simulink model "DCAC_conv_GFM"  (R2025a)
settings: Solver=VariableStepAuto  StartTime=0.0  StopTime=10.0  RelTol=1e-3
undefined symbols (not defined in the file): block_buses_DC, block_idx, Grid_op_VCVSC, Kic, Kiv, Kpc, Kpv, Nbuses_DC, op_VCVSC
libraries: simulink x6
(part 1 of 2)
settings Model: Creator=atomas  LastModifiedBy=atomas

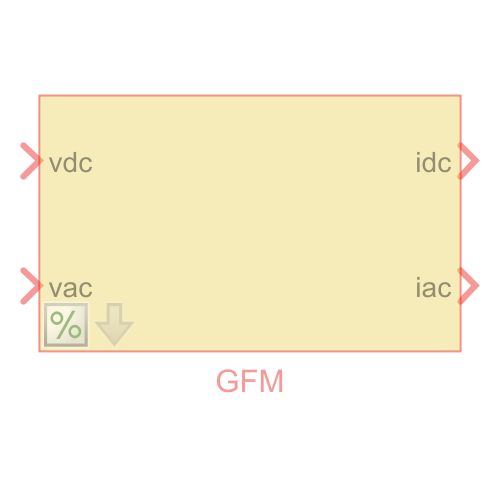
[thumbnail: Simulink's stored preview of the top-level diagram]
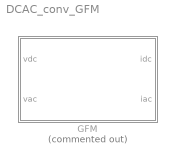
== system DCAC_conv_GFM ==
  GFM : Subsystem  Commented=on  mask(VCVSC){Pmax=Inf, Qmax=Inf, fb=50, dynamic_VCC=Static, Lf=0.01, Rf=0.001, Rcf=1000000, Cfi=0.1, Kint=1, Tint=0.1, Bint=1, Kext=1, Bext=1, Text=0.1, Fi=1, Tf=0.01, mp=0.01, nq=0.01, VI_L=0.1, VI_R=0.01, WOF_Tf=0, cf=0.1, cv=0.1, L_out=0.1, R_out=0.01}
      mask prompts: Pmax "Active power limit (p.u.)"; Qmax "Reactive power limit (p.u.)"; fb "Base frequency (Hz)"; dynamic_VCC "Dynamic behavior"; Lf "Filter inductance (pu)"; Rf "Filter resistance (pu)"; Rcf "Parallel resistance to C (pu)"; Cfi "Filter capacitance (pu)"; Fi "Current feedfordward gain"; Tf "Low-pass filter time constant (s)"; mp "Droop coefficient mp (pu)"; nq "Droop coefficient nq (pu)"; VI_L "Inductance (pu)"; VI_R "Resistance (pu)"; WOF_Tf "WOF time constant (s)"; cf "Frequency SC gain"; cv "Voltage SC gain"; L_out "Output inductance (p.u.)"; R_out "Output resistance (p.u.)"
      mask help: Grid-forming converter. VCC are the voltage and current controllers. Dynamic behavior includes the PI controllers, decoupling, current feedfordward and LC output filter. Static behavior consists of setting the reference voltage directly in the output. PC is the power controller including the droop control and low-pass filters for the power measurements.
      mask init:
      | mdlWks = get_param(bdroot,'ModelWorkspace'); % Get the model workspace
      | block_name = get_param(gcb,'Name');
      | bvarname = get_param(get_param(get_param(get_param(...
      |         gcb, 'Parent'), 'Parent'), 'Parent'), 'bvarname');
      | DC = mdlWks.getVariable([bvarname 'DC']);
      | try
      |     block_DC_buses = DC.(block_name + "s_DC_buses");
      |     block_buses = DC.(block_name + "s_buses");
      |     block_DC_toM = DC.(block_name + "s_DC_toM");
      |     block_toM = DC.(block_name + "s_toM");
      |     dparams = DC.(block_name + "_dparams");
      | catch ME
      |     %errordlg(ME.message)
      | end
      mask Help: web('Documentation/VCVSC.html')
      mask TypeOptions dynamic_VCC: Dynamic with limitation | Dynamic | Static | Dynamic VC and static CC
      mask Callback dynamic_VCC:
      | block = gcb;
      | dynamic = get_param(block, 'dynamic_VCC');
      | param_vis = get_param(block,'MaskVisibilities');
      | block_params = string(fieldnames(get_param(block, 'DialogParameters')));
      | switch dynamic
      |     case 'Dynamic'
      |         param_vis(find(block_params == 'Lf'):find(block_params == 'Fi')) = cellstr("on");
      |         set_param([gcb '/VCC'], 'LabelModeActiveChoice', 'dynamic');
      |     case 'Dynamic with limitation'
      |         param_vis(find(block_params == 'Lf'):find(block_params == 'Fi')) = cellstr("on");
      |         set_param([gcb '/VCC'], 'LabelModeActiveChoice', 'dynamic_limiting');
      |     case 'Static'
      |         param_vis(find(block_params == 'Lf'):find(block_params == 'Fi')) = cellstr("off");
      |         set_param([gcb '/VCC'], 'LabelModeActiveChoice', 'static');
      |     case 'Dynamic VC and static CC'
      |         param_vis(find(block_params == 'Lf'):find(block_params == 'Fi')) = cellstr("on");
      |         param_vis(ismember(block_params, ["Lf","Rf","Kpc","Kic","Fi"])) = cellstr("off");
      |         set_param([gcb '/VCC'], 'LabelModeActiveChoice', 'dynamic_VC');
      | end
      | set_param(block,'MaskVisibilities',param_vis)
      mask TypeOptions Tf: PC/Tf
      mask TypeOptions mp: PC/mp
      mask TypeOptions nq: PC/nq
      mask TypeOptions VI_L: VI/L
      mask TypeOptions VI_R: VI/R
      mask TypeOptions WOF_Tf: VI/Tf
      mask DialogControl Container8 Prompt: Parameters
      mask DialogControl VCC Prompt: VCC
      mask DialogControl PC Prompt: PC
      mask DialogControl VI Prompt: VI
      mask DialogControl SC Prompt: SC
      mask DialogControl Container9 Prompt: Others

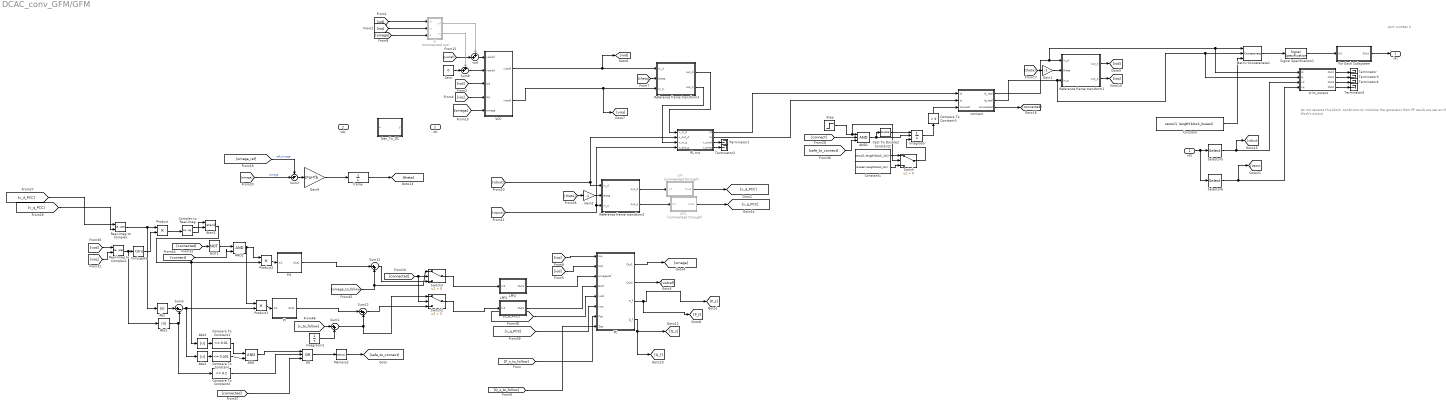
== system DCAC_conv_GFM/GFM ==
  note: do not rename this block, conditions to initialise the generator from PF result are set on this block's output
  note: port number 2
  vac : Inport
  vdc : Inport  Port=2
  AND : Logic  IconShape=distinctive  AllPortsSameDT=off  OutDataTypeStr=boolean
  AND1 : Logic  Inputs=3  IconShape=distinctive  AllPortsSameDT=off  OutDataTypeStr=boolean
  AND2 : Logic  IconShape=distinctive  AllPortsSameDT=off  OutDataTypeStr=boolean
  Abs{,1..3} (4 alike) : Abs  ZeroCross=off  SaturateOnIntegerOverflow=off
  Atan2 : Trigonometry  Operator=atan2
  Cast To Double2 : DataTypeConversion  OutDataTypeStr=double  SaturateOnIntegerOverflow=off  RndMeth=Floor
  Compare To Constant : simulink/Logic and Bit Operations/Compare To Constant  relop=<=  const=0.001  OutDataTypeStr=boolean  ZeroCross=off
  Compare To Constant1 : simulink/Logic and Bit Operations/Compare To Constant  relop=<=  const=0.01  OutDataTypeStr=boolean  ZeroCross=off
  Compare To Constant2 : simulink/Logic and Bit Operations/Compare To Constant  relop=<=  const=0.2  OutDataTypeStr=boolean  ZeroCross=off
  Compare To Constant3 : simulink/Logic and Bit Operations/Compare To Constant  relop=>  const=4  OutDataTypeStr=boolean  ZeroCross=off
  Complex to Real-Imag : ComplexToRealImag
  Conjugate : Math  Operator=conj  SignedPower=on  RndMeth=Zero
  Constant : Constant  Value=zeros(1, length(block_buses))  VectorParams1D=off
  Constant1 : Constant  Value=5*ones(1,length(block_idx))  VectorParams1D=off
  Constant2 : Constant  Value=zeros(1,length(block_idx))  VectorParams1D=off
  For Each Subsystem : Subsystem  TreatAsAtomicUnit=on
  Gain1 : Gain  Gain=-1
  Gain2 : Gain  Gain=-1
  Gain6 : Gain  Gain=2*pi*fb
  Gen_To_DC : MATLAB Function  TreatAsAtomicUnit=on
  Integrator : Integrator  ExternalReset=falling  InitialConditionSource=external  InitialCondition=Grid_op_VCVSC.States(1,:)
  Integrator1 : Integrator  InitialCondition=Grid_op_VCVSC.States(2,:)
  LPF : Subsystem  Commented=through
  LPF1 : Subsystem  Commented=through
  LPF2 : Subsystem
  LPF3 : Subsystem
  Matrix Concatenate1 : Concatenate  NumInputs=3  Mode=Multidimensional array
  Memory2 : Memory  InitialCondition=1
  NOT1 : Logic  Operator=NOT  IconShape=distinctive  AllPortsSameDT=off  OutDataTypeStr=boolean
  OR : Logic  Operator=OR  Inputs=3  IconShape=distinctive  AllPortsSameDT=off  OutDataTypeStr=boolean
  PC : Subsystem  mask(PC_VCVSC){Tf=Tf, mp=mp, nq=nq}
      mask prompts: Tf "Low-pass filter time constant (s)"; mp "Droop coefficient mp"; nq "Droop coefficient nq"
      mask help: Power controller of a grid-forming converter, including the droop control and low-pass filters for the power measurements.
      mask init:
      | if all(Tf ~= 0)
      |     iTf = 1./Tf;
      |     set_param([gcb '/LPF_P'],'Commented','off')
      |     set_param([gcb '/LPF_Q'],'Commented','off')
      | else
      |     set_param([gcb '/LPF_P'],'Commented','through')
      |     set_param([gcb '/LPF_Q'],'Commented','through')
      | end
  PI : Subsystem
  PI1 : Subsystem
  Product : Product
  Product1 : Product  OutDataTypeStr=double
  Product2 : Product  OutDataTypeStr=double
  RL out : Subsystem  Variant=on  VariantControlMode=label  LabelModeActiveChoice=dynamic  mask{dynamic=Dynamic, R=R_out, L=L_out, fbase=50}
      mask prompts: dynamic "Dynamic behavior"; R "Series resistance (p.u.)"; L "Inductance (p.u.)"; fbase "Base frequency (Hz)"
      mask init:
      | omegab = 2*pi*fbase;
      | invL = 1./L;
      | vssBlk = gcb;
      | switch dynamic
      |     case "Static"
      |         set_param(vssBlk, 'LabelModeActiveChoice', 'static');
      |     case "Dynamic"
      |         set_param(vssBlk, 'LabelModeActiveChoice', 'dynamic');
      |     case "Static omega"
      |         set_param(vssBlk, 'LabelModeActiveChoice', 'static_omega');
      | end
      mask TypeOptions dynamic: Static | Dynamic | Static omega
  Real-Imag to Complex : RealImagToComplex
  Real-Imag to Complex1 : RealImagToComplex
  Reference frame transform1 : Subsystem
  Reference frame transform2 : Subsystem
  Reference frame transform3 : Subsystem
  Selector5 : Selector  NumberOfDimensions=2  InputPortWidth=3  IndexOptions=Index vector (dialog),Index vector (dialog)  Indices=1,block_buses  OutputSizes=1,1
  Selector6 : Selector  NumberOfDimensions=2  InputPortWidth=3  IndexOptions=Index vector (dialog),Index vector (dialog)  Indices=2,block_buses  OutputSizes=1,1
  Signal Specification1 : SignalSpecification  Dimensions=[3 length(block_buses)]
  Step : Step  Time=0.01  SampleTime=0  VectorParams1D=off  ZeroCross=off
  Sum1 : Sum  Inputs=|++
  Sum11 : Sum  Inputs=|++
  Sum12 : Sum  Inputs=|++
  Sum2 : Sum  Inputs=-+|
  Sum3 : Sum  Inputs=|+-
  Sum8 : Sum  Inputs=++|
  Switch : Switch  Criteria=u2 > Threshold  SaturateOnIntegerOverflow=off  InputSameDT=off
  Switch2 : Switch  Criteria=u2 > Threshold  SaturateOnIntegerOverflow=off  InputSameDT=off
  Switch3 : Switch  Criteria=u2 > Threshold  SaturateOnIntegerOverflow=off  InputSameDT=off
  Terminator{,1..5} (6 alike) : Terminator
  VCC : Subsystem  Variant=on  VariantControlMode=label  LabelModeActiveChoice=static
  VI : Subsystem  Commented=on  mask{L=VI_L, R=VI_R, Tf=WOF_Tf}
      mask prompts: L "Inductance (pu)"; R "Resistance (pu)"; Tf "WOF time constant (s)"
      mask init:
      | if all(Tf ~= 0)
      |     iTf = 1./Tf;
      |     set_param([gcb '/WOF_d'],'Commented','off')
      |     set_param([gcb '/WOF_q'],'Commented','off')
      | else
      |     set_param([gcb '/WOF_d'],'Commented','through')
      |     set_param([gcb '/WOF_q'],'Commented','through')
      | end
  Zero : Constant  Value=0  OutDataTypeStr=Inherit: Inherit via back propagation
  connect : Subsystem
  frame : Integrator  InitialCondition=Grid_op_VCVSC.States(19,:)  IgnoreLimit=on
  trim_output : Subsystem
  vod : Sum  Inputs=++|
  iac : Outport
  idc : Outport  Port=2
  wires:
  Sum8/1 -> VCC/2(voqref)
  vod/1 -> VCC/1(vodref)
  [omega] -> VI/3(omega)
  [ioq] -> VI/2(iq)
  [iod] -> VI/1(id)
  Gain2/1 -> Reference frame transform2/2(theta)
  [theta] -> Gain2/1
  Gain6/1 -> frame/1
  frame/1 -> [theta]
  PC/4(Q_f) -> [Q_s], [Q_f]
  PC/3(P_f) -> [P_s], [P_f]
  connect/3(connected) -> [connected]
  [omega] -> Sum2/2  "omega"
  [omega_ref] -> Sum2/1  "ref_omega"
  Sum2/1 -> Gain6/1
  RL out/1(id) -> connect/1(id)
  [theta] -> Gain1/1
  Gain1/1 -> Reference frame transform1/2(theta)
  [ioq] -> VCC/4(ioq)
  [iod] -> VCC/3(iod)
  Zero/1 -> Sum8/2
  [vodref] -> vod/2
  [omega] -> VCC/5(omega)
  [theta] -> Reference frame transform3/2(theta)
  PC/1(Out1) -> [omega]
  PC/2(Out2) -> [vodref]
  [iod] -> PC/2(iodi)
  [ioq] -> PC/1(ioq)
  Reference frame transform1/2(out_q) -> [ioq]
  Reference frame transform3/1(out_d) -> RL out/1(v_in_d)
  Reference frame transform3/2(out_q) -> RL out/3(v_in_q)
  RL out/2(iq) -> connect/2(iq)
  Reference frame transform1/1(out_d) -> [iod]
  VI/1(vd) -> vod/1
  VI/2(vq) -> Sum8/1
  connect/1(id_real) -> trim_output/1(id), Matrix Concatenate1/1, Reference frame transform1/1(in_d)
  connect/2(iq_real) -> trim_output/2(iq), Matrix Concatenate1/2, Reference frame transform1/3(in_q)
  RL out/3(v_outd) -> Terminator1/1
  RL out/4(v_outq) -> Terminator2/1
  Reference frame transform2/1(out_d) -> LPF/1(In1)
  Reference frame transform2/2(out_q) -> LPF1/1(In1)
  [v_d_PCC] -> Real-Imag to Complex/1
  [v_q_PCC] -> Real-Imag to Complex/2
  [vod] -> Real-Imag to Complex1/1
  [voq] -> Real-Imag to Complex1/2
  Real-Imag to Complex1/1 -> Abs1/1, Conjugate/1
  Real-Imag to Complex/1 -> Abs/1, Product/1
  Conjugate/1 -> Product/2
  Product/1 -> Complex to Real-Imag/1
  Complex to Real-Imag/2 -> Atan2/1
  Complex to Real-Imag/1 -> Atan2/2
  Abs/1 -> Sum3/1
  Sum3/1 -> Abs2/1, Product1/2
  Product1/1 -> PI/1(In1)
  Product2/1 -> PI1/1(In1)
  Atan2/1 -> Abs3/1, Product2/2
  Abs1/1 -> Compare To Constant2/1, Sum3/2
  Abs2/1 -> Compare To Constant/1
  Compare To Constant/1 -> AND/2
  Abs3/1 -> Compare To Constant1/1
  Compare To Constant1/1 -> AND/1
  AND/1 -> OR/1
  OR/1 -> Memory2/1
  Compare To Constant2/1 -> OR/2
  [connected] -> OR/3
  Memory2/1 -> [safe_to_connect]
  [vqout] -> Reference frame transform2/3(in_q), RL out/4(v_out_q)
  LPF/1(Out1) -> [v_d_PCC]
  LPF1/1(Out1) -> [v_q_PCC]
  [vdout] -> RL out/2(v_out_d), Reference frame transform2/1(in_d)
  Matrix Concatenate1/1 -> Signal Specification1/1
  Constant/1 -> Matrix Concatenate1/3
  For Each Subsystem/1(Out1) -> iac/1
  Signal Specification1/1 -> For Each Subsystem/1(In1)
  [v_d_PCC] -> PC/5(vodi)
  [v_q_PCC] -> PC/6(voq)
  trim_output/1(Out1) -> Terminator/1
  trim_output/2(Out2) -> Terminator3/1
  trim_output/3(Out3) -> Terminator4/1
  trim_output/4(Out4) -> Terminator5/1
  vac/1 -> Selector6/1, Selector5/1
  Selector6/1 -> [vqout], trim_output/4(vq)
  Selector5/1 -> [vdout], trim_output/3(vd)
  NOT1/1 -> AND2/1
  [connected] -> NOT1/1
  AND2/1 -> Product1/1, Product2/1
  [connect] -> AND1/2
  Integrator/1 -> Compare To Constant3/1
  Constant2/1 -> Switch/1
  Step/1 -> Switch/2, AND1/1
  Constant1/1 -> Switch/3
  [safe_to_connect] -> AND1/3
  AND1/1 -> Cast To Double2/1, Integrator/2
  Cast To Double2/1 -> Integrator/1
  Switch/1 -> Integrator/3
  VCC/1(vidref) -> [vod], Reference frame transform3/1(in_d)
  VCC/2(viqref) -> [voq], Reference frame transform3/3(in_q)
  Sum12/1 -> Switch2/3
  Sum1/1 -> Switch2/1, Sum12/2
  [omega_to_follow] -> Sum11/2, Switch3/1
  [connected] -> Switch2/2, Switch3/2
  PI/1(Out1) -> Sum12/1
  PI1/1(Out1) -> Sum11/1
  Sum11/1 -> Switch3/3
  Switch3/1 -> LPF2/1(In1)
  Switch2/1 -> LPF3/1(In1)
  [P_s_to_follow] -> PC/7(Psp)
  [Q_s_to_follow] -> PC/8(Qsp)
  [v_to_follow] -> Sum1/1
  Integrator1/1 -> Sum1/2
  Compare To Constant3/1 -> connect/3(connect)
  [connect] -> AND2/2
  LPF2/1(Out1) -> PC/3(omegaref)
  LPF3/1(Out1) -> PC/4(Eref)

== system DCAC_conv_GFM/GFM/For Each Subsystem ==
  In1 : Inport  Partition=on  PartitionDimension=1  PartitionWidth=1  PartitionOffset=0
  For Each : ForEach  DisableCoverage=on
  State-Space : StateSpace  A=[]  B=[]  C=[]  D=block_toM  InitialCondition=0  ParameterTunability=Optimized
  Transpose : Math  Operator=transpose
  Transpose1 : Math  Operator=transpose
  Out1 : Outport  ConcatenationDimension=1
  wires:
  State-Space/1 -> Transpose1/1
  Transpose/1 -> State-Space/1
  Transpose1/1 -> Out1/1
  In1/1 -> Transpose/1

== system DCAC_conv_GFM/GFM/LPF ==
  In1 : Inport
  Gain : Gain  Gain=1e2
  I : Integrator  InitialCondition=Grid_op_VCVSC.op.States(4).x'
  Sum4 : Sum  Inputs=|+-
  Out1 : Outport
  wires:
  Gain/1 -> I/1
  Sum4/1 -> Gain/1
  In1/1 -> Sum4/1
  I/1 -> Out1/1, Sum4/2

== system DCAC_conv_GFM/GFM/LPF1 ==
  In1 : Inport
  Gain : Gain  Gain=1e2
  I : Integrator  InitialCondition=Grid_op_VCVSC.op.States(5).x'
  Sum4 : Sum  Inputs=|+-
  Out1 : Outport
  wires:
  I/1 -> Sum4/2, Out1/1
  In1/1 -> Sum4/1
  Sum4/1 -> Gain/1
  Gain/1 -> I/1

== system DCAC_conv_GFM/GFM/LPF2 ==
  In1 : Inport
  Gain : Gain  Gain=1e2
  I : Integrator  InitialCondition=Grid_op_VCVSC.States(3,:)
  Sum4 : Sum  Inputs=|+-
  Out1 : Outport
  wires:
  I/1 -> Sum4/2, Out1/1
  In1/1 -> Sum4/1
  Sum4/1 -> Gain/1
  Gain/1 -> I/1

== system DCAC_conv_GFM/GFM/LPF3 ==
  In1 : Inport
  Gain : Gain  Gain=1e2
  I : Integrator  InitialCondition=Grid_op_VCVSC.States(4,:)
  Sum4 : Sum  Inputs=|+-
  Out1 : Outport
  wires:
  Gain/1 -> I/1
  Sum4/1 -> Gain/1
  In1/1 -> Sum4/1
  I/1 -> Out1/1, Sum4/2

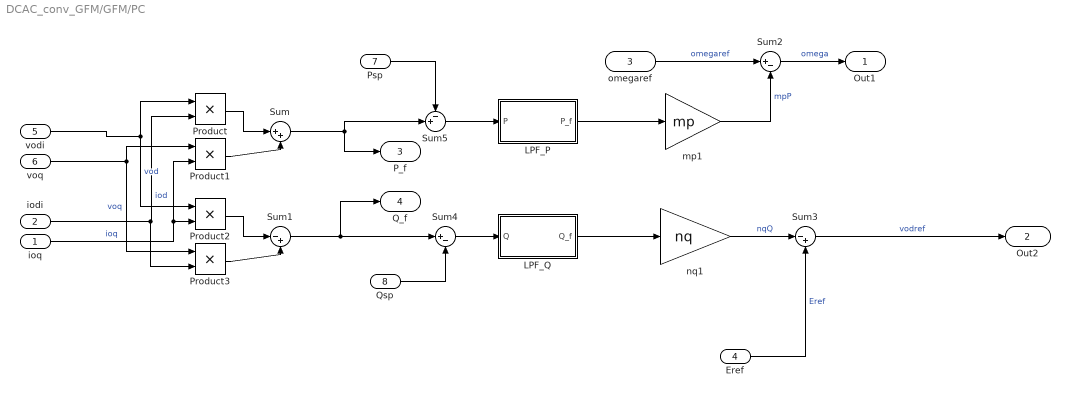
== system DCAC_conv_GFM/GFM/PC ==
  ioq : Inport
  iodi : Inport  Port=2
  omegaref : Inport  Port=3
  Eref : Inport  Port=4
  vodi : Inport  Port=5
  voq : Inport  Port=6
  Psp : Inport  Port=7
  Qsp : Inport  Port=8
  LPF_P : Subsystem
  LPF_Q : Subsystem
  Product{,1..3} (4 alike) : Product
  Sum : Sum  Inputs=|++
  Sum1 : Sum  Inputs=|-+
  Sum2 : Sum  Inputs=|+-
  Sum3 : Sum  Inputs=|-+
  Sum4 : Sum  Inputs=|+-
  Sum5 : Sum  Inputs=-+|
  mp1 : Gain  Gain=mp
  nq1 : Gain  Gain=nq
  Out1 : Outport
  Out2 : Outport  Port=2
  P_f : Outport  Port=3
  Q_f : Outport  Port=4
  wires:
  Sum2/1 -> Out1/1  "omega"
  vodi/1 -> Product2/1, Product/1  "vod"
  Product/1 -> Sum/1
  Product1/1 -> Sum/2
  Product2/1 -> Sum1/1
  Product3/1 -> Sum1/2
  nq1/1 -> Sum3/1  "nqQ"
  Eref/1 -> Sum3/2  "Eref"
  omegaref/1 -> Sum2/1  "omegaref"
  Sum/1 -> Sum5/2, P_f/1
  Sum1/1 -> Q_f/1, Sum4/1
  mp1/1 -> Sum2/2  "mpP"
  voq/1 -> Product1/1, Product3/1  "voq"
  iodi/1 -> Product3/2, Product/2  "iod"
  ioq/1 -> Product2/2, Product1/2  "ioq"
  Qsp/1 -> Sum4/2
  Sum4/1 -> LPF_Q/1(Q)
  Psp/1 -> Sum5/1
  Sum5/1 -> LPF_P/1(P)
  Sum3/1 -> Out2/1  "vodref"
  LPF_P/1(P_f) -> mp1/1
  LPF_Q/1(Q_f) -> nq1/1

== system DCAC_conv_GFM/GFM/PI ==
  In1 : Inport
  Gain : Gain  Gain=0.1
  Gain1 : Gain  Gain=0.2
  I : Integrator  InitialCondition=Grid_op_VCVSC.States(7,:)
  Sum10 : Sum  Inputs=|++
  Out1 : Outport
  wires:
  Gain1/1 -> I/1
  I/1 -> Sum10/2
  Gain/1 -> Sum10/1
  Sum10/1 -> Out1/1
  In1/1 -> Gain/1, Gain1/1

== system DCAC_conv_GFM/GFM/PI1 ==
  In1 : Inport
  Gain : Gain  Gain=0.1/100/pi
  Gain1 : Gain  Gain=0.2/100/pi
  I : Integrator  InitialCondition=Grid_op_VCVSC.States(8,:)
  Sum10 : Sum  Inputs=|++
  Out1 : Outport
  wires:
  In1/1 -> Gain1/1, Gain/1
  Sum10/1 -> Out1/1
  Gain/1 -> Sum10/1
  I/1 -> Sum10/2
  Gain1/1 -> I/1

== system DCAC_conv_GFM/GFM/RL out ==
  note: 1) Add Subsystem or Model blocks as valid variant choices.
      | 2) You cannot connect blocks at this level. At simulation, connectivity is automatically
      | determined, based on the active variant and port name matching.
  v_in_d : Inport
  v_out_d : Inport  Port=2
  v_in_q : Inport  Port=3
  v_out_q : Inport  Port=4
  dynamic : Subsystem  VariantControl=dynamic
  static : Subsystem  VariantControl=static
  static_omega : Subsystem  VariantControl=static_omega
  id : Outport
  iq : Outport  Port=2
  v_outd : Outport  Port=3
  v_outq : Outport  Port=4

== system DCAC_conv_GFM/GFM/Reference frame transform1 ==
  in_d : Inport
  theta : Inport  Port=2
  in_q : Inport  Port=3
  Complex to Real-Imag : ComplexToRealImag
  Cos : Trigonometry  SCDEnableBlockLinearizationSpecification=on  Operator=cos
  Product : Product
  Real-Imag to Complex : RealImagToComplex
  Real-Imag to Complex1 : RealImagToComplex
  Sin : Trigonometry  SCDEnableBlockLinearizationSpecification=on
  out_d : Outport
  out_q : Outport  Port=2
  wires:
  Complex to Real-Imag/2 -> out_q/1
  Real-Imag to Complex1/1 -> Product/1
  Real-Imag to Complex/1 -> Product/2
  Product/1 -> Complex to Real-Imag/1
  theta/1 -> Sin/1, Cos/1
  Cos/1 -> Real-Imag to Complex1/1
  Sin/1 -> Real-Imag to Complex1/2
  Complex to Real-Imag/1 -> out_d/1
  in_q/1 -> Real-Imag to Complex/2
  in_d/1 -> Real-Imag to Complex/1

== system DCAC_conv_GFM/GFM/Reference frame transform2 ==
  in_d : Inport
  theta : Inport  Port=2
  in_q : Inport  Port=3
  Complex to Real-Imag : ComplexToRealImag
  Cos : Trigonometry  SCDEnableBlockLinearizationSpecification=on  Operator=cos
  Product : Product
  Real-Imag to Complex : RealImagToComplex
  Real-Imag to Complex1 : RealImagToComplex
  Sin : Trigonometry  SCDEnableBlockLinearizationSpecification=on
  out_d : Outport
  out_q : Outport  Port=2
  wires:
  in_d/1 -> Real-Imag to Complex/1
  in_q/1 -> Real-Imag to Complex/2
  Complex to Real-Imag/1 -> out_d/1
  Sin/1 -> Real-Imag to Complex1/2
  Cos/1 -> Real-Imag to Complex1/1
  theta/1 -> Cos/1, Sin/1
  Product/1 -> Complex to Real-Imag/1
  Real-Imag to Complex/1 -> Product/2
  Real-Imag to Complex1/1 -> Product/1
  Complex to Real-Imag/2 -> out_q/1

== system DCAC_conv_GFM/GFM/Reference frame transform3 ==
  in_d : Inport
  theta : Inport  Port=2
  in_q : Inport  Port=3
  Complex to Real-Imag : ComplexToRealImag
  Cos : Trigonometry  SCDEnableBlockLinearizationSpecification=on  Operator=cos
  Product : Product
  Real-Imag to Complex : RealImagToComplex
  Real-Imag to Complex1 : RealImagToComplex
  Sin : Trigonometry  SCDEnableBlockLinearizationSpecification=on
  out_d : Outport
  out_q : Outport  Port=2
  wires:
  Complex to Real-Imag/2 -> out_q/1
  Real-Imag to Complex1/1 -> Product/1
  Real-Imag to Complex/1 -> Product/2
  Product/1 -> Complex to Real-Imag/1
  theta/1 -> Cos/1, Sin/1
  Cos/1 -> Real-Imag to Complex1/1
  Sin/1 -> Real-Imag to Complex1/2
  Complex to Real-Imag/1 -> out_d/1
  in_q/1 -> Real-Imag to Complex/2
  in_d/1 -> Real-Imag to Complex/1

== system DCAC_conv_GFM/GFM/VCC ==
  note: 1) Add Subsystem or Model blocks as valid variant choices.
      | 2) You cannot connect blocks at this level. At simulation, connectivity is automatically
      | determined, based on the active variant and port name matching.
  vodref : Inport
  voqref : Inport  Port=2
  iod : Inport  Port=3
  ioq : Inport  Port=4
  omega : Inport  Port=5
  dynamic : Subsystem  VariantControl=dynamic
  dynamic_VC : Subsystem  VariantControl=dynamic_VC
  dynamic_limiting : Subsystem  VariantControl=dynamic_limiting
  static : Subsystem  VariantControl=static
  vidref : Outport
  viqref : Outport  Port=2

== system DCAC_conv_GFM/GFM/VI ==
  id : Inport
  iq : Inport  Port=2
  omega : Inport  Port=3
  Gain : Gain  Gain=L
  Gain1 : Gain  Gain=R
  Gain2 : Gain  Gain=L
  Gain3 : Gain  Gain=R
  Product : Product
  Product1 : Product
  Sum : Sum  Inputs=-+|
  Sum1 : Sum  Inputs=|--
  WOF_d : Subsystem  Commented=through
  WOF_q : Subsystem  Commented=through
  vd : Outport
  vq : Outport  Port=2
  wires:
  WOF_q/1(Out1) -> Gain/1, Gain3/1
  WOF_d/1(Out1) -> Gain1/1, Gain2/1
  Sum1/1 -> vq/1
  Sum/1 -> vd/1
  Gain3/1 -> Sum1/2
  Gain1/1 -> Sum/1
  Product1/1 -> Sum1/1
  Gain2/1 -> Product1/2
  id/1 -> WOF_d/1(In1)
  Product/1 -> Sum/2
  iq/1 -> WOF_q/1(In1)
  omega/1 -> Product1/1, Product/2
  Gain/1 -> Product/1

== system DCAC_conv_GFM/GFM/connect ==
  id : Inport
  iq : Inport  Port=2
  connect : Inport  Port=3
  Switch : Switch  Criteria=u2 > Threshold  ZeroCross=off  SaturateOnIntegerOverflow=off  InputSameDT=off
  Switch1 : Switch  Criteria=u2 > Threshold  ZeroCross=off  SaturateOnIntegerOverflow=off  InputSameDT=off
  Zero1 : Constant  Value=0  VectorParams1D=off  OutDataTypeStr=Inherit: Inherit via back propagation
  Zero2 : Constant  Value=0  VectorParams1D=off  OutDataTypeStr=Inherit: Inherit via back propagation
  id_real : Outport
  iq_real : Outport  Port=2
  connected : Outport  Port=3  OutDataTypeStr=boolean
  wires:
  Switch/1 -> id_real/1
  Zero1/1 -> Switch/3
  id/1 -> Switch/1
  connect/1 -> connected/1, Switch1/2, Switch/2
  Switch1/1 -> iq_real/1
  iq/1 -> Switch1/1
  Zero2/1 -> Switch1/3

== system DCAC_conv_GFM/GFM/trim_output ==
  id : Inport
  iq : Inport  Port=2
  vd : Inport  Port=3
  vq : Inport  Port=4
  Out1 : Outport
  Out2 : Outport  Port=2
  Out3 : Outport  Port=3
  Out4 : Outport  Port=4
  wires:
  id/1 -> Out1/1
  vq/1 -> Out4/1
  vd/1 -> Out3/1
  iq/1 -> Out2/1

== system DCAC_conv_GFM/GFM/PC/LPF_P ==
  P : Inport
  Gain : Gain  Gain=iTf
  I : Integrator  InitialCondition=Grid_op_VCVSC.States(5,:)
  Sum4 : Sum  Inputs=|+-
  P_f : Outport
  wires:
  Gain/1 -> I/1
  Sum4/1 -> Gain/1
  P/1 -> Sum4/1
  I/1 -> P_f/1, Sum4/2

== system DCAC_conv_GFM/GFM/PC/LPF_Q ==
  Q : Inport
  Gain : Gain  Gain=iTf
  I : Integrator  InitialCondition=Grid_op_VCVSC.States(6,:)
  Sum4 : Sum  Inputs=|+-
  Q_f : Outport
  wires:
  Gain/1 -> I/1
  Q/1 -> Sum4/1
  I/1 -> Q_f/1, Sum4/2
  Sum4/1 -> Gain/1

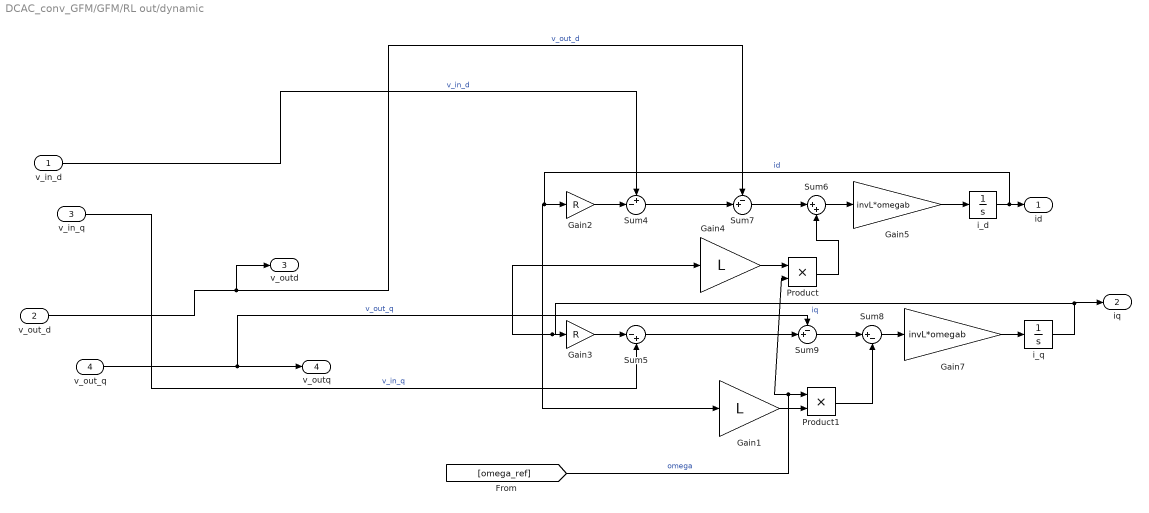
== system DCAC_conv_GFM/GFM/RL out/dynamic ==
  v_in_d : Inport
  v_out_d : Inport  Port=2
  v_in_q : Inport  Port=3
  v_out_q : Inport  Port=4
  Gain1 : Gain  Gain=L
  Gain2 : Gain  Gain=R
  Gain3 : Gain  Gain=R
  Gain4 : Gain  Gain=L
  Gain5 : Gain  Gain=invL*omegab
  Gain7 : Gain  Gain=invL*omegab
  Product : Product
  Product1 : Product
  Sum4 : Sum  Inputs=+-|
  Sum5 : Sum  Inputs=|-+
  Sum6 : Sum  Inputs=|++
  Sum7 : Sum  Inputs=-+|
  Sum8 : Sum  Inputs=|+-
  Sum9 : Sum  Inputs=-+|
  i_d : Integrator  InitialCondition=Grid_op_VCVSC.States(9,:)
  i_q : Integrator  InitialCondition=Grid_op_VCVSC.States(10,:)
  id : Outport
  iq : Outport  Port=2
  v_outd : Outport  Port=3
  v_outq : Outport  Port=4
  wires:
  v_out_q/1 -> v_outq/1, Sum9/1  "v_out_q"
  v_out_d/1 -> v_outd/1, Sum7/1  "v_out_d"
  Sum9/1 -> Sum8/1
  Gain1/1 -> Product1/2
  i_q/1 -> iq/1, Gain4/1, Gain3/1  "iq"
  Gain7/1 -> i_q/1
  Sum5/1 -> Sum9/2
  Gain3/1 -> Sum5/1
  Sum7/1 -> Sum6/1
  Gain4/1 -> Product/1
  Product1/1 -> Sum8/2
  Sum4/1 -> Sum7/2
  Sum8/1 -> Gain7/1
  Product/1 -> Sum6/2
  Gain5/1 -> i_d/1
  [omega_ref] -> Product/2, Product1/1  "omega"
  Sum6/1 -> Gain5/1
  i_d/1 -> id/1, Gain1/1, Gain2/1  "id"
  Gain2/1 -> Sum4/2
  v_in_d/1 -> Sum4/1  "v_in_d"
  v_in_q/1 -> Sum5/2  "v_in_q"

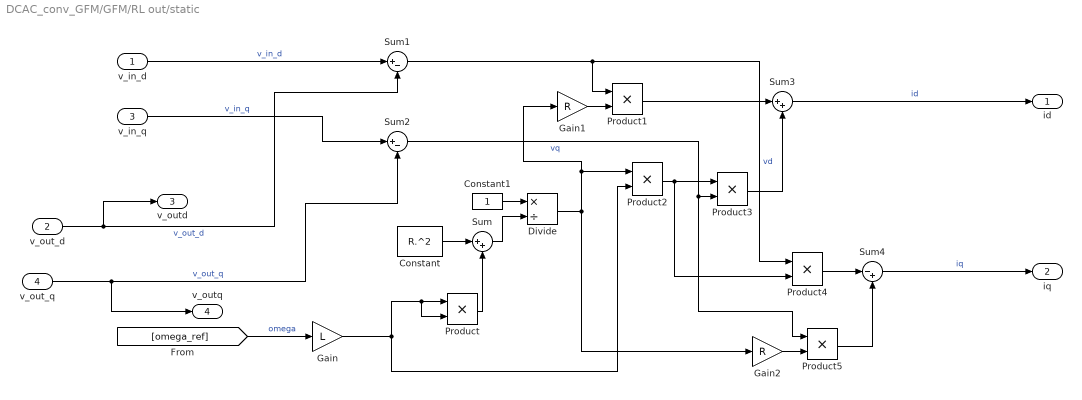
== system DCAC_conv_GFM/GFM/RL out/static ==
  v_in_d : Inport
  v_out_d : Inport  Port=2
  v_in_q : Inport  Port=3
  v_out_q : Inport  Port=4
  Constant : Constant  Value=R.^2
  Constant1 : Constant
  Divide : Product  Inputs=*/
  Gain : Gain  Gain=L
  Gain1 : Gain  Gain=R
  Gain2 : Gain  Gain=R
  Product{,1..5} (6 alike) : Product
  Sum : Sum  Inputs=|++
  Sum1 : Sum  Inputs=|+-
  Sum2 : Sum  Inputs=|+-
  Sum3 : Sum  Inputs=|++
  Sum4 : Sum  Inputs=|-+
  id : Outport
  iq : Outport  Port=2
  v_outd : Outport  Port=3
  v_outq : Outport  Port=4
  wires:
  [omega_ref] -> Gain/1  "omega"
  v_in_d/1 -> Sum1/1  "v_in_d"
  v_out_q/1 -> v_outq/1, Sum2/2  "v_out_q"
  Sum4/1 -> iq/1  "iq"
  Sum3/1 -> id/1  "id"
  Gain1/1 -> Product1/2
  Product2/1 -> Product4/2, Product3/1
  Product4/1 -> Sum4/1
  Divide/1 -> Gain2/1, Gain1/1, Product2/1
  Sum1/1 -> Product1/1, Product4/1  "vd"
  Product3/1 -> Sum3/2
  Constant1/1 -> Divide/1
  Gain/1 -> Product/2, Product/1, Product2/2
  Sum2/1 -> Product5/1, Product3/2  "vq"
  Constant/1 -> Sum/1
  Product5/1 -> Sum4/2
  Product1/1 -> Sum3/1
  Product/1 -> Sum/2
  Gain2/1 -> Product5/2
  Sum/1 -> Divide/2
  v_out_d/1 -> v_outd/1, Sum1/2  "v_out_d"
  v_in_q/1 -> Sum2/1  "v_in_q"

== system DCAC_conv_GFM/GFM/RL out/static_omega ==
  v_in_d : Inport
  v_out_d : Inport  Port=2
  v_in_q : Inport  Port=3
  v_out_q : Inport  Port=4
  Gain : Gain  Gain=1./(R.^2+L.^2)
  Gain2 : Gain  Gain=1./(R.^2+L.^2)
  Gain3 : Gain  Gain=R
  Gain4 : Gain  Gain=L
  Gain5 : Gain  Gain=L
  Gain6 : Gain  Gain=R
  Sum : Sum  Inputs=|++
  Sum1 : Sum  Inputs=|+-
  Sum2 : Sum  Inputs=|+-
  Sum3 : Sum  Inputs=|-+
  id : Outport
  iq : Outport  Port=2
  v_outd : Outport  Port=3
  v_outq : Outport  Port=4
  wires:
  v_in_q/1 -> Sum2/1  "v_in_q"
  v_in_d/1 -> Sum1/1  "v_in_d"
  v_out_q/1 -> v_outq/1, Sum2/2  "v_out_q"
  v_out_d/1 -> v_outd/1, Sum1/2  "v_out_d"
  Sum1/1 -> Gain/1  "vd"
  Sum2/1 -> Gain2/1  "vq"
  Gain/1 -> Gain5/1, Gain3/1
  Gain3/1 -> Sum/1
  Gain4/1 -> Sum/2
  Gain2/1 -> Gain6/1, Gain4/1
  Sum/1 -> id/1
  Gain5/1 -> Sum3/1
  Sum3/1 -> iq/1
  Gain6/1 -> Sum3/2

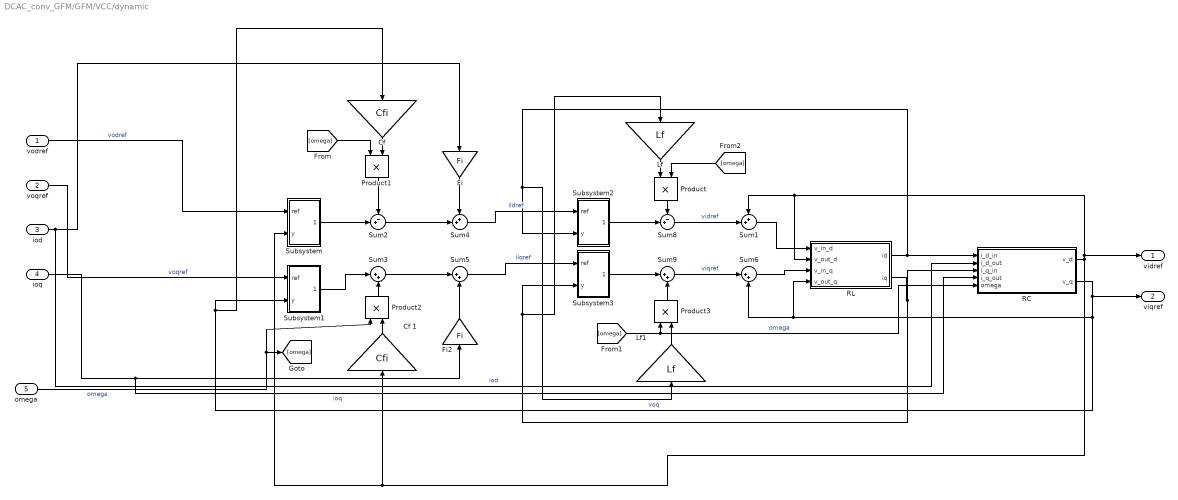
== system DCAC_conv_GFM/GFM/VCC/dynamic ==
  vodref : Inport
  voqref : Inport  Port=2
  iod : Inport  Port=3
  ioq : Inport  Port=4
  omega : Inport  Port=5
  Cf : Gain  Gain=Cfi
  Cf 1 : Gain  Gain=Cfi
  Fi : Gain  Gain=Fi
  Fi2 : Gain  Gain=Fi
  "Lf " : Gain  Gain=Lf
  Lf1 : Gain  Gain=Lf
  Product{,1..3} (4 alike) : Product
  RC : Subsystem  Variant=on  VariantControlMode=label  LabelModeActiveChoice=dynamic  mask{dynamic=Dynamic, R=Rcf, C=Cfi, fbase=50}
      mask prompts: dynamic "Dynamic behavior"; R "Parallel resistance (p.u.)"; C "Capacitance (p.u.)"; fbase "Base frequency (Hz)"
      mask init:
      | omegab = 2*pi*fbase;
      | iC = 1./C;
      | iR = 1./R;
      | vssBlk = gcb;
      | switch dynamic
      |     case "Dynamic"
      |         set_param(vssBlk, 'LabelModeActiveChoice', 'dynamic');
      |     case "Static"
      |         set_param(vssBlk, 'LabelModeActiveChoice', 'static');
      |     case "Static omega"
      |         set_param(vssBlk, 'LabelModeActiveChoice', 'static omega');
      | end
      mask TypeOptions dynamic: Dynamic | Static | Static omega
  RL : Subsystem  Variant=on  VariantControlMode=label  LabelModeActiveChoice=dynamic  mask(Line){dynamic=Dynamic, R=Rf, L=Lf, fbase=fb}
      mask prompts: dynamic "Dynamic behavior"; R "Series resistance (p.u.)"; L "Inductance (p.u.)"; fbase "Base frequency (Hz)"
      mask init: same as DCAC_conv_GFM/GFM/RL out
      mask Help: web('Documentation/RL.html')
      mask TypeOptions dynamic: Static | Dynamic | Static omega
  Subsystem : Subsystem
  Subsystem1 : Subsystem
  Subsystem2 : Subsystem
  Subsystem3 : Subsystem
  Sum1 : Sum  Inputs=++|
  Sum2 : Sum  Inputs=-+|
  Sum{3,5..6,9} (4 alike) : Sum  Inputs=|++
  Sum4 : Sum  Inputs=++|
  Sum8 : Sum  Inputs=-+|
  vidref : Outport
  viqref : Outport  Port=2
  wires:
  Sum5/1 -> Subsystem3/1(ref)  "ilqref"
  Product/1 -> Sum8/1
  vodref/1 -> Subsystem/1(ref)  "vodref"
  RC/2(v_q) -> viqref/1, Sum6/2, RL/4(v_out_q), Subsystem1/2(y), Cf/1  "voq"
  [omega] -> Product/2
  Lf1/1 -> Product3/2
  Fi/1 -> Sum4/1
  voqref/1 -> Subsystem1/1(ref)  "voqref"
  Product3/1 -> Sum9/2
  Product2/1 -> Sum3/2
  Cf 1/1 -> Product2/2
  Cf/1 -> Product1/2
  Sum4/1 -> Subsystem2/1(ref)  "ildref"
  Product1/1 -> Sum2/1
  iod/1 -> RC/2(i_d_out), Fi/1  "iod"
  Sum2/1 -> Sum4/2
  "Lf "/1 -> Product/1
  Sum3/1 -> Sum5/1
  [omega] -> RC/5(omega), Product3/1  "omega"
  ioq/1 -> RC/4(i_q_out), Fi2/1  "ioq"
  Fi2/1 -> Sum5/2
  Subsystem/1(Out1) -> Sum2/2
  Subsystem1/1(Out1) -> Sum3/1
  Subsystem2/1(Out1) -> Sum8/2
  Subsystem3/1(Out1) -> Sum9/1
  omega/1 -> Product2/1, [omega]  "omega"
  [omega] -> Product1/1
  RC/1(v_d) -> vidref/1, Sum1/1, RL/2(v_out_d), Subsystem/2(y), Cf 1/1
  RL/1(id) -> Subsystem2/2(y), Lf1/1, RC/1(i_d_in)
  RL/2(iq) -> RC/3(i_q_in), Subsystem3/2(y), "Lf "/1
  Sum8/1 -> Sum1/2  "vidref"
  Sum9/1 -> Sum6/1  "viqref"
  Sum1/1 -> RL/1(v_in_d)
  Sum6/1 -> RL/3(v_in_q)

== system DCAC_conv_GFM/GFM/VCC/dynamic_VC ==
  vodref : Inport
  voqref : Inport  Port=2
  iod : Inport  Port=3
  ioq : Inport  Port=4
  omega : Inport  Port=5
  Cf : Gain  Gain=Cfi
  Cf 1 : Gain  Gain=Cfi
  Fi : Gain  Gain=Fi
  Fi2 : Gain  Gain=Fi
  Product1 : Product
  Product2 : Product
  RC : Subsystem  Variant=on  VariantControlMode=label  LabelModeActiveChoice=dynamic  mask{dynamic=Dynamic, R=Rcf, C=Cfi, fbase=50}
      mask prompts: dynamic "Dynamic behavior"; R "Parallel resistance (p.u.)"; C "Capacitance (p.u.)"; fbase "Base frequency (Hz)"
      mask init: same as DCAC_conv_GFM/GFM/VCC/dynamic/RC
      mask TypeOptions dynamic: Dynamic | Static | Static omega
  Subsystem : Subsystem
  Subsystem1 : Subsystem
  Sum2 : Sum  Inputs=-+|
  Sum3 : Sum  Inputs=|++
  Sum4 : Sum  Inputs=++|
  Sum5 : Sum  Inputs=|++
  vidref : Outport
  viqref : Outport  Port=2
  wires:
  [omega] -> Product1/1
  omega/1 -> RC/5(omega), Product2/1, [omega]  "omega"
  Subsystem1/1(Out1) -> Sum3/1
  Subsystem/1(Out1) -> Sum2/2
  Fi2/1 -> Sum5/2
  ioq/1 -> RC/4(i_q_out), Fi2/1  "ioq"
  Sum3/1 -> Sum5/1
  Sum2/1 -> Sum4/2
  iod/1 -> RC/2(i_d_out), Fi/1  "iod"
  Product1/1 -> Sum2/1
  Cf/1 -> Product1/2
  Cf 1/1 -> Product2/2
  Product2/1 -> Sum3/2
  voqref/1 -> Subsystem1/1(ref)  "voqref"
  Fi/1 -> Sum4/1
  RC/2(v_q) -> viqref/1, Cf/1, Subsystem1/2(y)
  vodref/1 -> Subsystem/1(ref)  "vodref"
  RC/1(v_d) -> vidref/1, Cf 1/1, Subsystem/2(y)
  Sum4/1 -> RC/1(i_d_in)
  Sum5/1 -> RC/3(i_q_in)

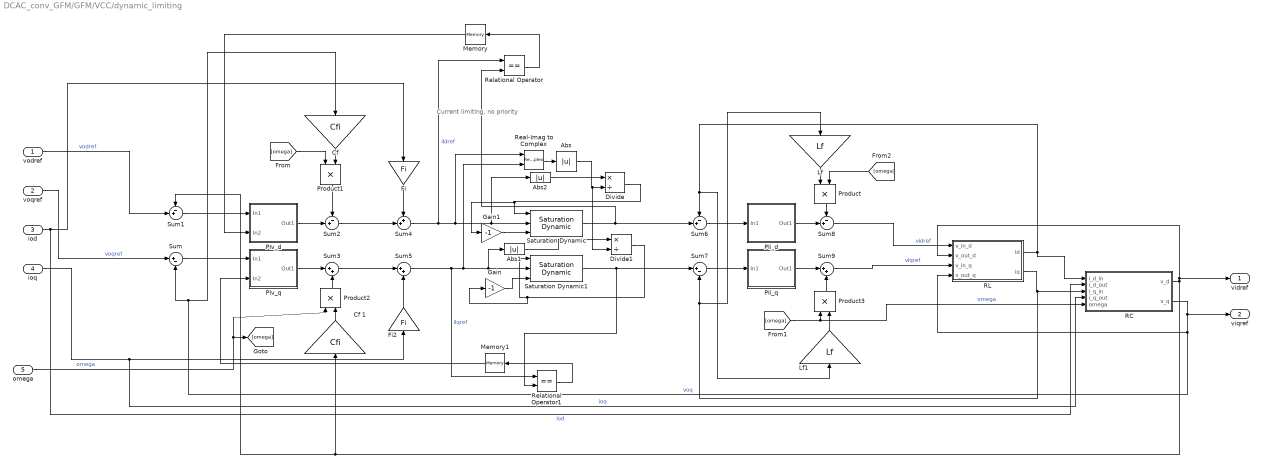
== system DCAC_conv_GFM/GFM/VCC/dynamic_limiting ==
  note: Current limiting, no priority
  vodref : Inport
  voqref : Inport  Port=2
  iod : Inport  Port=3
  ioq : Inport  Port=4
  omega : Inport  Port=5
  Abs : Abs  ZeroCross=off  SaturateOnIntegerOverflow=off
  Abs1 : Abs  ZeroCross=off  SaturateOnIntegerOverflow=off
  Abs2 : Abs  ZeroCross=off  SaturateOnIntegerOverflow=off
  Cf : Gain  Gain=Cfi
  Cf 1 : Gain  Gain=Cfi
  Divide : Product  Inputs=*/
  Divide1 : Product  Inputs=*/
  Fi : Gain  Gain=Fi
  Fi2 : Gain  Gain=Fi
  Gain : Gain  Gain=-1
  Gain1 : Gain  Gain=-1
  "Lf " : Gain  Gain=Lf
  Lf1 : Gain  Gain=Lf
  Memory : Memory  InitialCondition=1  LinearizeMemory=on
  Memory1 : Memory  InitialCondition=1  LinearizeMemory=on
  PIi_d : Subsystem
  PIi_q : Subsystem
  PIv_d : Subsystem
  PIv_q : Subsystem
  Product{,1..3} (4 alike) : Product
  RC : Subsystem  Variant=on  VariantControlMode=label  LabelModeActiveChoice=dynamic  mask{dynamic=Dynamic, R=Rcf, C=Cfi, fbase=50}
      mask prompts: dynamic "Dynamic behavior"; R "Parallel resistance (p.u.)"; C "Capacitance (p.u.)"; fbase "Base frequency (Hz)"
      mask init: same as DCAC_conv_GFM/GFM/VCC/dynamic/RC
      mask TypeOptions dynamic: Dynamic | Static | Static omega
  RL : Subsystem  Variant=on  VariantControlMode=label  LabelModeActiveChoice=dynamic  mask(Line){dynamic=Dynamic, R=Rf, L=Lf, fbase=fb}
      mask prompts: dynamic "Dynamic behavior"; R "Series resistance (p.u.)"; L "Inductance (p.u.)"; fbase "Base frequency (Hz)"
      mask init: same as DCAC_conv_GFM/GFM/RL out
      mask Help: web('Documentation/RL.html')
      mask TypeOptions dynamic: Static | Dynamic | Static omega
  Real-Imag to Complex : RealImagToComplex
  Relational Operator : RelationalOperator  Operator===  OutDataTypeStr=boolean  ZeroCross=off  RndMeth=Simplest  InputSameDT=off
  Relational Operator1 : RelationalOperator  Operator===  OutDataTypeStr=boolean  ZeroCross=off  RndMeth=Simplest  InputSameDT=off
  Saturation Dynamic : simulink/Discontinuities/Saturation Dynamic  OutMin=[]  OutMax=[]  OutDataTypeStr=Inherit: Same as second input  OutDataType=fixdt(1, 16)  OutScaling=2^-10  DoSatur=off
  Saturation Dynamic1 : simulink/Discontinuities/Saturation Dynamic  OutMin=[]  OutMax=[]  OutDataTypeStr=Inherit: Same as second input  OutDataType=fixdt(1, 16)  OutScaling=2^-10  DoSatur=off
  Sum : Sum  Inputs=|+-
  Sum{1..2,6,8} (4 alike) : Sum  Inputs=-+|
  Sum3 : Sum  Inputs=|++
  Sum4 : Sum  Inputs=++|
  Sum5 : Sum  Inputs=|++
  Sum7 : Sum  Inputs=|+-
  Sum9 : Sum  Inputs=|++
  vidref : Outport
  viqref : Outport  Port=2
  wires:
  Saturation Dynamic/1 -> Sum6/2, Relational Operator/2
  Saturation Dynamic1/1 -> Sum7/1, Relational Operator1/2
  Abs2/1 -> Divide/1
  Abs1/1 -> Divide1/1
  Sum9/1 -> RL/3(v_in_q)  "viqref"
  Sum8/1 -> RL/1(v_in_d)  "vidref"
  RL/2(iq) -> Sum7/2, "Lf "/1, RC/3(i_q_in)
  RL/1(id) -> RC/1(i_d_in), Sum6/1, Lf1/1
  RC/1(v_d) -> Sum1/1, Cf 1/1, RL/2(v_out_d), vidref/1
  [omega] -> Product1/1
  omega/1 -> [omega], Product2/1  "omega"
  PIi_q/1(Out1) -> Sum9/1
  PIi_d/1(Out1) -> Sum8/2
  PIv_q/1(Out1) -> Sum3/1
  PIv_d/1(Out1) -> Sum2/2
  Fi2/1 -> Sum5/2
  ioq/1 -> Fi2/1, RC/4(i_q_out)  "ioq"
  [omega] -> Product3/1, RC/5(omega)  "omega"
  Sum3/1 -> Sum5/1
  "Lf "/1 -> Product/1
  Sum7/1 -> PIi_q/1(In1)
  Sum2/1 -> Sum4/2
  iod/1 -> Fi/1, RC/2(i_d_out)  "iod"
  Product1/1 -> Sum2/1
  Sum4/1 -> Relational Operator/1, Abs2/1, Saturation Dynamic/2, Real-Imag to Complex/1  "ildref"
  Cf/1 -> Product1/2
  Cf 1/1 -> Product2/2
  Product2/1 -> Sum3/2
  Product3/1 -> Sum9/2
  voqref/1 -> Sum/1  "voqref"
  Sum6/1 -> PIi_d/1(In1)
  Fi/1 -> Sum4/1
  Lf1/1 -> Product3/2
  [omega] -> Product/2
  RC/2(v_q) -> Cf/1, Sum/2, RL/4(v_out_q), viqref/1  "voq"
  vodref/1 -> Sum1/2  "vodref"
  Product/1 -> Sum8/1
  Sum5/1 -> Relational Operator1/1, Abs1/1, Saturation Dynamic1/2, Real-Imag to Complex/2  "ilqref"
  Real-Imag to Complex/1 -> Abs/1
  Abs/1 -> Divide1/2, Divide/2
  Divide/1 -> Gain1/1, Saturation Dynamic/1
  Divide1/1 -> Gain/1, Saturation Dynamic1/1
  Gain/1 -> Saturation Dynamic1/3
  Gain1/1 -> Saturation Dynamic/3
  Sum1/1 -> PIv_d/1(In1)
  Relational Operator/1 -> Memory/1
  Sum/1 -> PIv_q/1(In1)
  Relational Operator1/1 -> Memory1/1
  Memory1/1 -> PIv_q/2(In2)
  Memory/1 -> PIv_d/2(In2)

== system DCAC_conv_GFM/GFM/VCC/static ==
  vodref : Inport
  voqref : Inport  Port=2
  iod : Inport  Port=3
  ioq : Inport  Port=4
  omega : Inport  Port=5
  Terminator : Terminator
  Terminator1 : Terminator
  Terminator2 : Terminator
  vidref : Outport
  viqref : Outport  Port=2
  wires:
  voqref/1 -> viqref/1  "voqref"
  vodref/1 -> vidref/1  "vodref"
  iod/1 -> Terminator/1  "iod"
  ioq/1 -> Terminator1/1  "ioq"
  omega/1 -> Terminator2/1  "ioq"

== system DCAC_conv_GFM/GFM/VI/WOF_d ==
  In1 : Inport
  Gain : Gain  Gain=iTf
  I : Integrator  InitialConditionSource=external  InitialCondition=Grid_op_VCVSC.op.States(6).x'
  Sum : Sum  Inputs=+-|
  Sum4 : Sum  Inputs=|+-
  Out1 : Outport
  wires:
  Sum/1 -> Out1/1
  I/1 -> Sum4/2, Sum/2
  In1/1 -> Sum4/1, Sum/1, I/2
  Sum4/1 -> Gain/1
  Gain/1 -> I/1

== system DCAC_conv_GFM/GFM/VI/WOF_q ==
  In1 : Inport
  Gain : Gain  Gain=iTf
  I : Integrator  InitialConditionSource=external  InitialCondition=Grid_op_VCVSC.op.States(7).x'
  Sum : Sum  Inputs=+-|
  Sum4 : Sum  Inputs=|+-
  Out1 : Outport
  wires:
  Sum/1 -> Out1/1
  I/1 -> Sum4/2, Sum/2
  In1/1 -> Sum4/1, Sum/1, I/2
  Sum4/1 -> Gain/1
  Gain/1 -> I/1

== system DCAC_conv_GFM/GFM/VCC/dynamic/RC ==
  note: 1) Add Subsystem or Model blocks as valid variant choices.
      | 2) You cannot connect blocks at this level. At simulation, connectivity is automatically
      | determined, based on the active variant and port name matching.
  i_d_in : Inport
  i_d_out : Inport  Port=2
  i_q_in : Inport  Port=3
  i_q_out : Inport  Port=4
  omega : Inport  Port=5
  dynamic : Subsystem  VariantControl=dynamic  mask{v_d_0=1}
      mask prompts: v_d_0 "Initial condition for v_d"
  static : Subsystem  VariantControl=static
  static omega : Subsystem  VariantControl=static omega
  v_d : Outport
  v_q : Outport  Port=2

== system DCAC_conv_GFM/GFM/VCC/dynamic/RL ==
  note: 1) Add Subsystem or Model blocks as valid variant choices.
      | 2) You cannot connect blocks at this level. At simulation, connectivity is automatically
      | determined, based on the active variant and port name matching.
  v_in_d : Inport
  v_out_d : Inport  Port=2
  v_in_q : Inport  Port=3
  v_out_q : Inport  Port=4
  dynamic : Subsystem  VariantControl=dynamic
      settings: PortSchema="{\"entries\":[{\"content\":{\"sides\":[{\"content\":{\"connectorIds\":[\"In1\"]},\"type\":\"ConnectorPlacement.EquallySpacedRectSide\",\"uuid\":\"63966e24-f9e7-4b2d-b456-7f4ea5e3f230\"},{\"content\":{\"connectorIds\":[\"In2\",\"In3\",\"In4\",\"Out1\",\"Out2\"],\"side\":\"RIGHT\"},\"type\":\"ConnectorPlacement.EquallySpacedRectSide\",\"uuid\":\"ded6ef04-52fd-47df-8e49-cf16b827098d\"},{\"content\":{\"connectorIds\":[],\"side\":\"TOP\"},\"type\":\"ConnectorPlacement.EquallySpacedRectSide\",\"uuid\":\"f940a985-fa23-4968-ad44-1d76d0e20c6a\"}]},\"type\":\"ConnectorPlacement.EquallySpacedConnector\",\"uuid\":\"20f61d3c-9af2-4982-98ea-af4910e61c9c\"}],\"packageUris\":[\"http://schema.mathworks.com/mf0/Connector/R2020b\"],\"version\":\"1.0\"}"
  static : Subsystem  VariantControl=static
  static_omega : Subsystem  VariantControl=static_omega
  id : Outport
  iq : Outport  Port=2

== system DCAC_conv_GFM/GFM/VCC/dynamic/Subsystem ==
  ref : Inport
  y : Inport  Port=2
  Gain : Gain  Gain=Bext
  Gain1 : Gain  Gain=1/Text
  Gain2 : Gain  Gain=Kext
  Integrator : Integrator  InitialCondition=Grid_op_VCVSC.States(15,:)
  Sum : Sum  Inputs=++|
  Sum1 : Sum  Inputs=|+-
  Sum6 : Sum  Inputs=|+-
  Out1 : Outport
  wires:
  y/1 -> Sum1/2, Sum6/2
  ref/1 -> Gain/1, Sum6/1
  Gain/1 -> Sum1/1
  Sum/1 -> Gain2/1
  Sum1/1 -> Sum/1
  Sum6/1 -> Gain1/1
  Gain1/1 -> Integrator/1
  Integrator/1 -> Sum/2
  Gain2/1 -> Out1/1

== system DCAC_conv_GFM/GFM/VCC/dynamic/Subsystem1 ==
  ref : Inport
  y : Inport  Port=2
  Gain : Gain  Gain=Bext
  Gain1 : Gain  Gain=1/Text
  Gain2 : Gain  Gain=Kext
  Integrator : Integrator  InitialCondition=Grid_op_VCVSC.States(16,:)
  Sum : Sum  Inputs=++|
  Sum1 : Sum  Inputs=|+-
  Sum6 : Sum  Inputs=|+-
  Out1 : Outport
  wires:
  Gain2/1 -> Out1/1
  Integrator/1 -> Sum/2
  Gain1/1 -> Integrator/1
  Sum6/1 -> Gain1/1
  Sum1/1 -> Sum/1
  Sum/1 -> Gain2/1
  Gain/1 -> Sum1/1
  ref/1 -> Sum6/1, Gain/1
  y/1 -> Sum6/2, Sum1/2

== system DCAC_conv_GFM/GFM/VCC/dynamic/Subsystem2 ==
  ref : Inport
  y : Inport  Port=2
  Gain : Gain  Gain=Bint
  Gain1 : Gain  Gain=1/Tint
  Gain2 : Gain  Gain=Kint
  Integrator : Integrator  InitialCondition=Grid_op_VCVSC.States(17,:)
  Sum : Sum  Inputs=++|
  Sum1 : Sum  Inputs=|+-
  Sum6 : Sum  Inputs=|+-
  Out1 : Outport
  wires:
  y/1 -> Sum1/2, Sum6/2
  ref/1 -> Gain/1, Sum6/1
  Gain/1 -> Sum1/1
  Sum/1 -> Gain2/1
  Sum1/1 -> Sum/1
  Sum6/1 -> Gain1/1
  Gain1/1 -> Integrator/1
  Integrator/1 -> Sum/2
  Gain2/1 -> Out1/1

== system DCAC_conv_GFM/GFM/VCC/dynamic/Subsystem3 ==
  ref : Inport
  y : Inport  Port=2
  Gain : Gain  Gain=Bint
  Gain1 : Gain  Gain=1/Tint
  Gain2 : Gain  Gain=Kint
  Integrator : Integrator  InitialCondition=Grid_op_VCVSC.States(18,:)
  Sum : Sum  Inputs=++|
  Sum1 : Sum  Inputs=|+-
  Sum6 : Sum  Inputs=|+-
  Out1 : Outport
  wires:
  Gain2/1 -> Out1/1
  Integrator/1 -> Sum/2
  Gain1/1 -> Integrator/1
  Sum6/1 -> Gain1/1
  Sum1/1 -> Sum/1
  Sum/1 -> Gain2/1
  Gain/1 -> Sum1/1
  ref/1 -> Sum6/1, Gain/1
  y/1 -> Sum6/2, Sum1/2

== system DCAC_conv_GFM/GFM/VCC/dynamic_VC/RC ==
  note: 1) Add Subsystem or Model blocks as valid variant choices.
      | 2) You cannot connect blocks at this level. At simulation, connectivity is automatically
      | determined, based on the active variant and port name matching.
  i_d_in : Inport
  i_d_out : Inport  Port=2
  i_q_in : Inport  Port=3
  i_q_out : Inport  Port=4
  omega : Inport  Port=5
  dynamic : Subsystem  VariantControl=dynamic  mask{v_d_0=1}
      mask prompts: v_d_0 "Initial condition for v_d"
  static : Subsystem  VariantControl=static
  static omega : Subsystem  VariantControl=static omega
  v_d : Outport
  v_q : Outport  Port=2

== system DCAC_conv_GFM/GFM/VCC/dynamic_VC/Subsystem ==
  ref : Inport
  y : Inport  Port=2
  Gain : Gain  Gain=Bext
  Gain1 : Gain  Gain=1/Text
  Gain2 : Gain  Gain=Kext
  Integrator : Integrator  InitialCondition=Grid_op_VCVSC.op.States(10).x'
  Sum : Sum  Inputs=++|
  Sum1 : Sum  Inputs=|+-
  Sum6 : Sum  Inputs=|+-
  Out1 : Outport
  wires:
  y/1 -> Sum1/2, Sum6/2
  ref/1 -> Gain/1, Sum6/1
  Gain/1 -> Sum1/1
  Sum/1 -> Gain2/1
  Sum1/1 -> Sum/1
  Sum6/1 -> Gain1/1
  Gain1/1 -> Integrator/1
  Integrator/1 -> Sum/2
  Gain2/1 -> Out1/1

== system DCAC_conv_GFM/GFM/VCC/dynamic_VC/Subsystem1 ==
  ref : Inport
  y : Inport  Port=2
  Gain : Gain  Gain=Bext
  Gain1 : Gain  Gain=1/Text
  Gain2 : Gain  Gain=Kext
  Integrator : Integrator  InitialCondition=Grid_op_VCVSC.op.States(11).x'
  Sum : Sum  Inputs=++|
  Sum1 : Sum  Inputs=|+-
  Sum6 : Sum  Inputs=|+-
  Out1 : Outport
  wires:
  Gain2/1 -> Out1/1
  Integrator/1 -> Sum/2
  Gain1/1 -> Integrator/1
  Sum6/1 -> Gain1/1
  Sum1/1 -> Sum/1
  Sum/1 -> Gain2/1
  Gain/1 -> Sum1/1
  ref/1 -> Sum6/1, Gain/1
  y/1 -> Sum6/2, Sum1/2

== system DCAC_conv_GFM/GFM/VCC/dynamic_limiting/PIi_d ==
  In1 : Inport
  Gain : Gain  Gain=Kpc
  Gain1 : Gain  Gain=Kic
  I : Integrator  InitialCondition=op_VCVSC.op.States(6).x'
  Sum10 : Sum  Inputs=|++
  Out1 : Outport
  wires:
  Gain1/1 -> I/1
  In1/1 -> Gain1/1, Gain/1
  Sum10/1 -> Out1/1
  Gain/1 -> Sum10/1
  I/1 -> Sum10/2

== system DCAC_conv_GFM/GFM/VCC/dynamic_limiting/PIi_q ==
  In1 : Inport
  Gain : Gain  Gain=Kpc
  Gain1 : Gain  Gain=Kic
  I : Integrator  InitialCondition=op_VCVSC.op.States(7).x'
  Sum10 : Sum  Inputs=|++
  Out1 : Outport
  wires:
  Gain1/1 -> I/1
  In1/1 -> Gain1/1, Gain/1
  Sum10/1 -> Out1/1
  Gain/1 -> Sum10/1
  I/1 -> Sum10/2

== system DCAC_conv_GFM/GFM/VCC/dynamic_limiting/PIv_d ==
  In1 : Inport
  In2 : Inport  Port=2
  Gain : Gain  Gain=Kpv
  Gain1 : Gain  Gain=Kiv
  I : Integrator  InitialCondition=op_VCVSC.op.States(8).x'
  Product : Product
  Sum10 : Sum  Inputs=|++
  Out1 : Outport
  wires:
  Gain1/1 -> Product/1
  In1/1 -> Gain1/1, Gain/1
  Sum10/1 -> Out1/1
  Gain/1 -> Sum10/1
  I/1 -> Sum10/2
  Product/1 -> I/1
  In2/1 -> Product/2

== system DCAC_conv_GFM/GFM/VCC/dynamic_limiting/PIv_q ==
  In1 : Inport
  In2 : Inport  Port=2
  Gain : Gain  Gain=Kpv
  Gain1 : Gain  Gain=Kiv
  I : Integrator  InitialCondition=op_VCVSC.op.States(9).x'
  Product : Product
  Sum10 : Sum  Inputs=|++
  Out1 : Outport
  wires:
  In2/1 -> Product/2
  Product/1 -> I/1
  I/1 -> Sum10/2
  Gain/1 -> Sum10/1
  Sum10/1 -> Out1/1
  In1/1 -> Gain/1, Gain1/1
  Gain1/1 -> Product/1

== system DCAC_conv_GFM/GFM/VCC/dynamic_limiting/RC ==
  note: 1) Add Subsystem or Model blocks as valid variant choices.
      | 2) You cannot connect blocks at this level. At simulation, connectivity is automatically
      | determined, based on the active variant and port name matching.
  i_d_in : Inport
  i_d_out : Inport  Port=2
  i_q_in : Inport  Port=3
  i_q_out : Inport  Port=4
  omega : Inport  Port=5
  dynamic : Subsystem  VariantControl=dynamic  mask{v_d_0=1}
      mask prompts: v_d_0 "Initial condition for v_d"
  static : Subsystem  VariantControl=static
  static omega : Subsystem  VariantControl=static omega
  v_d : Outport
  v_q : Outport  Port=2

== system DCAC_conv_GFM/GFM/VCC/dynamic_limiting/RL ==
  note: 1) Add Subsystem or Model blocks as valid variant choices.
      | 2) You cannot connect blocks at this level. At simulation, connectivity is automatically
      | determined, based on the active variant and port name matching.
  v_in_d : Inport
  v_out_d : Inport  Port=2
  v_in_q : Inport  Port=3
  v_out_q : Inport  Port=4
  dynamic : Subsystem  VariantControl=dynamic
      settings: PortSchema="{\"entries\":[{\"content\":{\"sides\":[{\"content\":{\"connectorIds\":[\"In1\"]},\"type\":\"ConnectorPlacement.EquallySpacedRectSide\",\"uuid\":\"63966e24-f9e7-4b2d-b456-7f4ea5e3f230\"},{\"content\":{\"connectorIds\":[\"In2\",\"In3\",\"In4\",\"Out1\",\"Out2\"],\"side\":\"RIGHT\"},\"type\":\"ConnectorPlacement.EquallySpacedRectSide\",\"uuid\":\"ded6ef04-52fd-47df-8e49-cf16b827098d\"},{\"content\":{\"connectorIds\":[],\"side\":\"TOP\"},\"type\":\"ConnectorPlacement.EquallySpacedRectSide\",\"uuid\":\"f940a985-fa23-4968-ad44-1d76d0e20c6a\"}]},\"type\":\"ConnectorPlacement.EquallySpacedConnector\",\"uuid\":\"20f61d3c-9af2-4982-98ea-af4910e61c9c\"}],\"packageUris\":[\"http://schema.mathworks.com/mf0/Connector/R2020b\"],\"version\":\"1.0\"}"
  static : Subsystem  VariantControl=static
  static_omega : Subsystem  VariantControl=static_omega
  id : Outport
  iq : Outport  Port=2

== system DCAC_conv_GFM/GFM/VCC/dynamic/RC/dynamic ==
  omega : Inport
  i_d_in : Inport  Port=2
  i_d_out : Inport  Port=3
  i_q_in : Inport  Port=4
  i_q_out : Inport  Port=5
  Gain1 : Gain  Gain=iR
  Gain2 : Gain  Gain=iR
  Gain3 : Gain  Gain=C
  Gain4 : Gain  Gain=C
  Gain5 : Gain  Gain=iC*omegab
  Gain6 : Gain  Gain=iC*omegab
  Product : Product
  Product1 : Product
  Sum10 : Sum  Inputs=|-++
  Sum11 : Sum  Inputs=-+|
  Sum12 : Sum  Inputs=|+-
  Sum13 : Sum  Inputs=-+-|
  vd : Integrator  InitialCondition=Grid_op_VCVSC.States(11,:)
  vq : Integrator  InitialCondition=Grid_op_VCVSC.States(12,:)
  v_d : Outport
  v_q : Outport  Port=2
  wires:
  Sum10/1 -> Gain6/1
  Gain3/1 -> Product1/1
  vq/1 -> v_q/1, Gain2/1, Gain3/1  "vq"
  Product1/1 -> Sum10/3
  Gain4/1 -> Product/1
  Gain2/1 -> Sum13/3
  Product/1 -> Sum13/1
  Sum11/1 -> Sum10/2
  Gain6/1 -> vd/1
  omega/1 -> Product/2, Product1/2  "omega"
  Sum13/1 -> Gain5/1
  Gain1/1 -> Sum10/1
  Gain5/1 -> vq/1
  Sum12/1 -> Sum13/2
  vd/1 -> Gain4/1, v_d/1, Gain1/1  "vd"
  i_d_in/1 -> Sum11/2  "id1"
  i_d_out/1 -> Sum11/1  "id2"
  i_q_in/1 -> Sum12/1  "iq1"
  i_q_out/1 -> Sum12/2  "iq2"

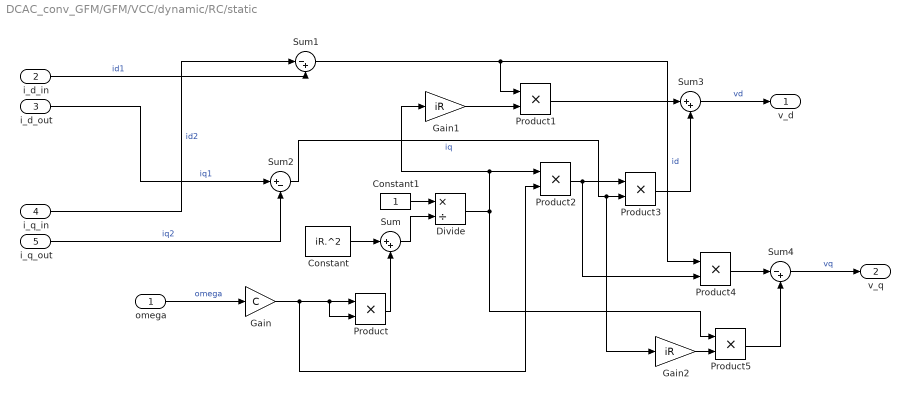
== system DCAC_conv_GFM/GFM/VCC/dynamic/RC/static ==
  omega : Inport
  i_d_in : Inport  Port=2
  i_d_out : Inport  Port=3
  i_q_in : Inport  Port=4
  i_q_out : Inport  Port=5
  Constant : Constant  Value=iR.^2
  Constant1 : Constant
  Divide : Product  Inputs=*/
  Gain : Gain  Gain=C
  Gain1 : Gain  Gain=iR
  Gain2 : Gain  Gain=iR
  Product{,1..5} (6 alike) : Product
  Sum : Sum  Inputs=|++
  Sum1 : Sum  Inputs=|-+
  Sum2 : Sum  Inputs=|+-
  Sum3 : Sum  Inputs=|++
  Sum4 : Sum  Inputs=|-+
  v_d : Outport
  v_q : Outport  Port=2
  wires:
  Product5/1 -> Sum4/2
  Gain2/1 -> Product5/2
  Product4/1 -> Sum4/1
  Product2/1 -> Product3/1, Product4/2
  Product3/1 -> Sum3/2
  Product1/1 -> Sum3/1
  Divide/1 -> Product2/1, Gain1/1, Product5/1
  Gain1/1 -> Product1/2
  Sum2/1 -> Product3/2, Gain2/1  "iq"
  Sum1/1 -> Product4/1, Product1/1  "id"
  Constant1/1 -> Divide/1
  Product/1 -> Sum/2
  Gain/1 -> Product/1, Product/2, Product2/2
  Sum/1 -> Divide/2
  Constant/1 -> Sum/1
  Sum4/1 -> v_q/1  "vq"
  Sum3/1 -> v_d/1  "vd"
  omega/1 -> Gain/1  "omega"
  i_d_in/1 -> Sum1/2  "id1"
  i_q_in/1 -> Sum1/1  "id2"
  i_d_out/1 -> Sum2/1  "iq1"
  i_q_out/1 -> Sum2/2  "iq2"

== system DCAC_conv_GFM/GFM/VCC/dynamic/RC/static omega ==
  i_d_in : Inport
  i_d_out : Inport  Port=2
  i_q_in : Inport  Port=3
  i_q_out : Inport  Port=4
  Gain : Gain  Gain=1./(iR.^2+C.^2)
  Gain2 : Gain  Gain=1./(iR.^2+C.^2)
  Gain3 : Gain  Gain=iR
  Gain4 : Gain  Gain=C
  Gain5 : Gain  Gain=iR
  Gain6 : Gain  Gain=C
  Sum : Sum  Inputs=|++
  Sum1 : Sum  Inputs=|+-
  Sum2 : Sum  Inputs=|+-
  Sum4 : Sum  Inputs=|-+
  v_d : Outport
  v_q : Outport  Port=2
  wires:
  i_q_in/1 -> Sum2/1  "iq1"
  Sum1/1 -> Gain/1  "id"
  Sum2/1 -> Gain2/1  "iq"
  i_q_out/1 -> Sum2/2  "iq2"
  i_d_in/1 -> Sum1/1  "id"
  i_d_out/1 -> Sum1/2
  Gain/1 -> Gain4/1, Gain3/1
  Gain2/1 -> Gain6/1, Gain5/1
  Gain3/1 -> Sum/1
  Gain6/1 -> Sum/2
  Gain4/1 -> Sum4/1
  Gain5/1 -> Sum4/2
  Sum4/1 -> v_q/1
  Sum/1 -> v_d/1
